simulink library "lib_BuildingThermalTL"  (R2026a)
settings: Solver=VariableStepAuto
libraries: ExternalWall_lib x47, WallSelector_lib x36, fl_lib x20, RoomWithRadiatorAndUFP x15, RoomLevelControl_lib x2
(part 1 of 5)
settings Model: Creator=vikrants  LastModifiedBy=vikrants

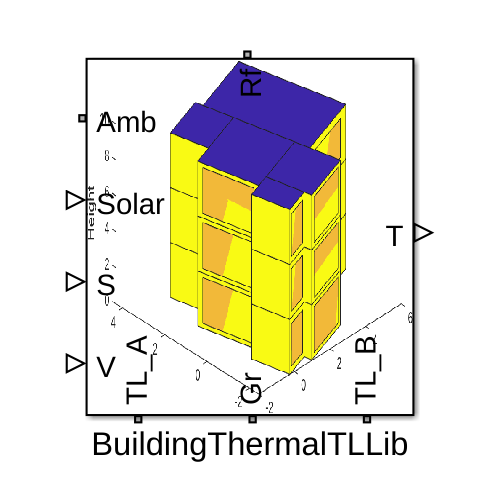
[thumbnail: Simulink's stored preview of the top-level diagram]
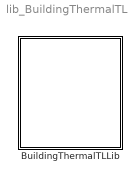
== system lib_BuildingThermalTL ==
  BuildingThermalTLLib : Subsystem
      settings: PortSchema="{\"entries\":[{\"content\":{\"sides\":[{\"content\":{\"connectorIds\":[\"LConn1\",\"LConn2\",\"LConn3\",\"LConn4\"]},\"type\":\"ConnectorPlacement.EquallySpacedRectSide\",\"uuid\":\"7752f6df-96a7-479d-81d0-a1acc354bc8e\"},{\"content\":{\"connectorIds\":[\"RConn1\"],\"side\":\"RIGHT\"},\"type\":\"ConnectorPlacement.EquallySpacedRectSide\",\"uuid\":\"82977a39-da32-427b-b825-91d4f4b46228\"},{\"content\":{\"connectorIds\":[\"LConn5\"],\"side\":\"TOP\"},\"type\":\"ConnectorPlacement.EquallySpacedRectSide\",\"uuid\":\"1009c293-c44e-4703-95e9-5e2b8b92121f\"},{\"content\":{\"connectorIds\":[\"RConn2\",\"RConn3\",\"RConn4\"],\"side\":\"BOTTOM\"},\"type\":\"ConnectorPlacement.EquallySpacedRectSide\",\"uuid\":\"f5115ea0-1536-4578-9315-a120045d60b6\"}]},\"type\":\"ConnectorPlacement.EquallySpacedConnector\",\"uuid\":\"9ddcc19a-e483-4977-a29d-e666927a4fbb\"}],\"packageUris\":[\"http://schema.mathworks.com/mf0/Connector/R2020b\"],\"version\":\"1.0\"}"
      mask Display: image('lib_BuildingThermalTL.png')

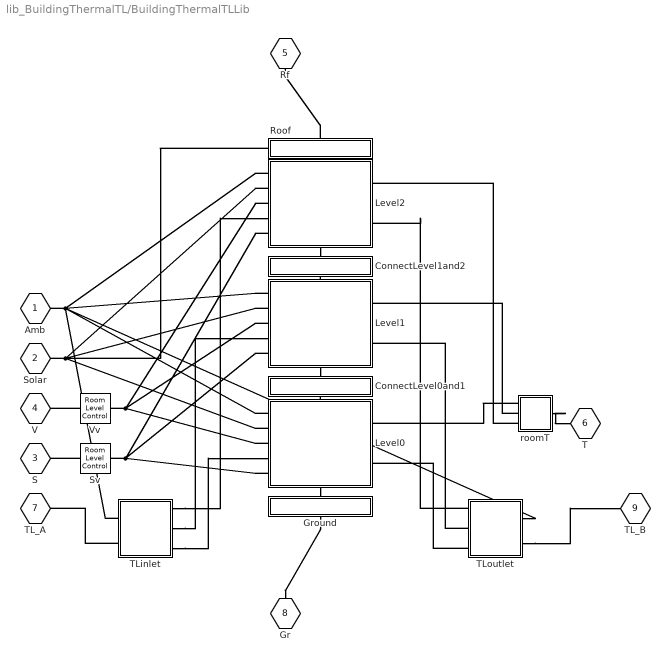
== system lib_BuildingThermalTL/BuildingThermalTLLib ==
  ConnectLevel0and1 : Subsystem
      settings: PortSchema="{\"entries\":[{\"content\":{\"sides\":[{\"content\":{},\"type\":\"ConnectorPlacement.EquallySpacedRectSide\",\"uuid\":\"bfcbcdaf-7e68-43ba-b21b-739e3d917df2\"},{\"content\":{\"side\":\"RIGHT\"},\"type\":\"ConnectorPlacement.EquallySpacedRectSide\",\"uuid\":\"1db46710-465c-454f-9fe4-f8c04c90b155\"},{\"content\":{\"connectorIds\":[\"LConn1\"],\"side\":\"TOP\"},\"type\":\"ConnectorPlacement.EquallySpacedRectSide\",\"uuid\":\"8ba3322a-28ec-4bcd-a32b-78c0e69bc71f\"},{\"content\":{\"connectorIds\":[\"RConn1\"],\"side\":\"BOTTOM\"},\"type\":\"ConnectorPlacement.EquallySpacedRectSide\",\"uuid\":\"deed2508-d6b6-4274-ba05-c274e079ee5b\"}]},\"type\":\"ConnectorPlacement.EquallySpacedConnector\",\"uuid\":\"bc7fd7cc-de66-4685-913a-91b57874b9ec\"}],\"packageUris\":[\"http://schema.mathworks.com/mf0/Connector/R2020b\"],\"version\":\"1.0\"}"
  ConnectLevel1and2 : Subsystem
      settings: PortSchema="{\"entries\":[{\"content\":{\"sides\":[{\"content\":{},\"type\":\"ConnectorPlacement.EquallySpacedRectSide\",\"uuid\":\"bfcbcdaf-7e68-43ba-b21b-739e3d917df2\"},{\"content\":{\"side\":\"RIGHT\"},\"type\":\"ConnectorPlacement.EquallySpacedRectSide\",\"uuid\":\"1db46710-465c-454f-9fe4-f8c04c90b155\"},{\"content\":{\"connectorIds\":[\"LConn1\"],\"side\":\"TOP\"},\"type\":\"ConnectorPlacement.EquallySpacedRectSide\",\"uuid\":\"8ba3322a-28ec-4bcd-a32b-78c0e69bc71f\"},{\"content\":{\"connectorIds\":[\"RConn1\"],\"side\":\"BOTTOM\"},\"type\":\"ConnectorPlacement.EquallySpacedRectSide\",\"uuid\":\"a3884e5a-d735-4cb4-ba23-284eb55af6b2\"}]},\"type\":\"ConnectorPlacement.EquallySpacedConnector\",\"uuid\":\"bc7fd7cc-de66-4685-913a-91b57874b9ec\"}],\"packageUris\":[\"http://schema.mathworks.com/mf0/Connector/R2020b\"],\"version\":\"1.0\"}"
  Ground : Subsystem
      settings: PortSchema="{\"entries\":[{\"content\":{\"sides\":[{\"content\":{},\"type\":\"ConnectorPlacement.EquallySpacedRectSide\",\"uuid\":\"bfcbcdaf-7e68-43ba-b21b-739e3d917df2\"},{\"content\":{\"side\":\"RIGHT\"},\"type\":\"ConnectorPlacement.EquallySpacedRectSide\",\"uuid\":\"1db46710-465c-454f-9fe4-f8c04c90b155\"},{\"content\":{\"connectorIds\":[\"LConn1\"],\"side\":\"TOP\"},\"type\":\"ConnectorPlacement.EquallySpacedRectSide\",\"uuid\":\"8ba3322a-28ec-4bcd-a32b-78c0e69bc71f\"},{\"content\":{\"connectorIds\":[\"RConn1\"],\"side\":\"BOTTOM\"},\"type\":\"ConnectorPlacement.EquallySpacedRectSide\",\"uuid\":\"62f17525-a3e4-4f49-87ca-4f069149a482\"}]},\"type\":\"ConnectorPlacement.EquallySpacedConnector\",\"uuid\":\"bc7fd7cc-de66-4685-913a-91b57874b9ec\"}],\"packageUris\":[\"http://schema.mathworks.com/mf0/Connector/R2020b\"],\"version\":\"1.0\"}"
  Level0 : Subsystem
      settings: PortSchema="{\"entries\":[{\"content\":{\"sides\":[{\"content\":{\"connectorIds\":[\"LConn1\",\"LConn2\",\"LConn3\",\"LConn4\",\"LConn5\"]},\"type\":\"ConnectorPlacement.EquallySpacedRectSide\",\"uuid\":\"deabb5b8-c24f-48fb-93fe-496ddd92a6f5\"},{\"content\":{\"connectorIds\":[\"RConn1\",\"RConn2\"],\"side\":\"RIGHT\"},\"type\":\"ConnectorPlacement.EquallySpacedRectSide\",\"uuid\":\"554b1cd5-3627-4990-b424-868f4b09881c\"},{\"content\":{\"connectorIds\":[\"LConn6\"],\"side\":\"TOP\"},\"type\":\"ConnectorPlacement.EquallySpacedRectSide\",\"uuid\":\"21e43258-e745-4398-91f3-d3fef9b84a06\"},{\"content\":{\"connectorIds\":[\"RConn3\"],\"side\":\"BOTTOM\"},\"type\":\"ConnectorPlacement.EquallySpacedRectSide\",\"uuid\":\"c4a37077-5805-4bd2-bf9a-83a9fce6d671\"}]},\"type\":\"ConnectorPlacement.EquallySpacedConnector\",\"uuid\":\"65daea52-a8f7-4065-b13d-a48c2b26414b\"}],\"packageUris\":[\"http://schema.mathworks.com/mf0/Connector/R2020b\"],\"version\":\"1.0\"}"
  Level1 : Subsystem
      settings: PortSchema="{\"entries\":[{\"content\":{\"sides\":[{\"content\":{\"connectorIds\":[\"LConn1\",\"LConn2\",\"LConn3\",\"LConn4\",\"LConn5\"]},\"type\":\"ConnectorPlacement.EquallySpacedRectSide\",\"uuid\":\"deabb5b8-c24f-48fb-93fe-496ddd92a6f5\"},{\"content\":{\"connectorIds\":[\"RConn1\",\"RConn2\"],\"side\":\"RIGHT\"},\"type\":\"ConnectorPlacement.EquallySpacedRectSide\",\"uuid\":\"554b1cd5-3627-4990-b424-868f4b09881c\"},{\"content\":{\"connectorIds\":[\"LConn6\"],\"side\":\"TOP\"},\"type\":\"ConnectorPlacement.EquallySpacedRectSide\",\"uuid\":\"21e43258-e745-4398-91f3-d3fef9b84a06\"},{\"content\":{\"connectorIds\":[\"RConn3\"],\"side\":\"BOTTOM\"},\"type\":\"ConnectorPlacement.EquallySpacedRectSide\",\"uuid\":\"0cd4818a-d5ce-48ab-9e4b-3620ed85a804\"}]},\"type\":\"ConnectorPlacement.EquallySpacedConnector\",\"uuid\":\"65daea52-a8f7-4065-b13d-a48c2b26414b\"}],\"packageUris\":[\"http://schema.mathworks.com/mf0/Connector/R2020b\"],\"version\":\"1.0\"}"
  Level2 : Subsystem
      settings: PortSchema="{\"entries\":[{\"content\":{\"sides\":[{\"content\":{\"connectorIds\":[\"LConn1\",\"LConn2\",\"LConn3\",\"LConn4\",\"LConn5\"]},\"type\":\"ConnectorPlacement.EquallySpacedRectSide\",\"uuid\":\"deabb5b8-c24f-48fb-93fe-496ddd92a6f5\"},{\"content\":{\"connectorIds\":[\"RConn1\",\"RConn2\"],\"side\":\"RIGHT\"},\"type\":\"ConnectorPlacement.EquallySpacedRectSide\",\"uuid\":\"554b1cd5-3627-4990-b424-868f4b09881c\"},{\"content\":{\"connectorIds\":[\"LConn6\"],\"side\":\"TOP\"},\"type\":\"ConnectorPlacement.EquallySpacedRectSide\",\"uuid\":\"21e43258-e745-4398-91f3-d3fef9b84a06\"},{\"content\":{\"connectorIds\":[\"RConn3\"],\"side\":\"BOTTOM\"},\"type\":\"ConnectorPlacement.EquallySpacedRectSide\",\"uuid\":\"b1810ee7-4d08-40c9-8b26-724c07e39c34\"}]},\"type\":\"ConnectorPlacement.EquallySpacedConnector\",\"uuid\":\"65daea52-a8f7-4065-b13d-a48c2b26414b\"}],\"packageUris\":[\"http://schema.mathworks.com/mf0/Connector/R2020b\"],\"version\":\"1.0\"}"
  Roof : Subsystem
      settings: PortSchema="{\"entries\":[{\"content\":{\"sides\":[{\"content\":{\"connectorIds\":[\"LConn1\"]},\"type\":\"ConnectorPlacement.EquallySpacedRectSide\",\"uuid\":\"330a1f4c-788b-45d3-8144-461e13e4bc2b\"},{\"content\":{\"side\":\"RIGHT\"},\"type\":\"ConnectorPlacement.EquallySpacedRectSide\",\"uuid\":\"2ff68f0e-d161-486d-a47e-10633b293a9f\"},{\"content\":{\"connectorIds\":[\"LConn2\"],\"side\":\"TOP\"},\"type\":\"ConnectorPlacement.EquallySpacedRectSide\",\"uuid\":\"a18254b5-007e-4575-8004-ea2058ac2122\"},{\"content\":{\"connectorIds\":[\"RConn1\"],\"side\":\"BOTTOM\"},\"type\":\"ConnectorPlacement.EquallySpacedRectSide\",\"uuid\":\"b51dbafe-ebd1-4fa9-aca1-0d2d3d6d1c44\"}]},\"type\":\"ConnectorPlacement.EquallySpacedConnector\",\"uuid\":\"c0f19b20-ad71-4ed9-8cf3-6c486454730f\"}],\"packageUris\":[\"http://schema.mathworks.com/mf0/Connector/R2020b\"],\"version\":\"1.0\"}"
  Sv : RoomLevelControl_lib/Room Level Control  portOption=roomControlOption.heat  roomMapping=[1 1 1 1;1 1 2 2;1 1 3 3;1 1 4 4;1 1 5 5;2 2 1 6;2 2 2 7;2 2 3 8;2 2 4 9;2 2 5 10;3 3 1 11;3 3 2 12;3 3 3 13;3 3 4 14;3 3 5 15]
  TLinlet : Subsystem
  TLoutlet : Subsystem
  Vv : RoomLevelControl_lib/Room Level Control  portOption=roomControlOption.valve  roomMapping=[1 1 1 1;1 1 2 2;1 1 3 3;1 1 4 4;1 1 5 5;2 2 1 6;2 2 2 7;2 2 3 8;2 2 4 9;2 2 5 10;3 3 1 11;3 3 2 12;3 3 3 13;3 3 4 14;3 3 5 15]
  roomT : Subsystem
  Amb : PMIOPort  Side=Left
  Solar : PMIOPort  Port=2  Side=Left
  S : PMIOPort  Port=3  Side=Left
  V : PMIOPort  Port=4  Side=Left
  Rf : PMIOPort  Port=5  Side=Left
  T : PMIOPort  Port=6  Side=Right
  TL_A : PMIOPort  Port=7  Side=Right
  Gr : PMIOPort  Port=8  Side=Right
  TL_B : PMIOPort  Port=9  Side=Right
  connections:
  TLinlet/RConn1 -- Level2/LConn4
  TLoutlet/LConn1 -- Level2/RConn2
  TLinlet/RConn2 -- Level1/LConn4
  TLoutlet/LConn2 -- Level1/RConn2
  TLinlet/RConn3 -- Level0/LConn4
  TLoutlet/LConn3 -- Level0/RConn2
  Level0/RConn3 -- Ground/LConn1
  Level1/RConn3 -- ConnectLevel0and1/LConn1
  Level0/LConn6 -- ConnectLevel0and1/RConn1
  Level2/RConn3 -- ConnectLevel1and2/LConn1
  Level1/LConn6 -- ConnectLevel1and2/RConn1
  Level2/LConn6 -- Roof/RConn1
  Sv/LConn1 -- S/RConn1
  Vv/LConn1 -- V/RConn1
  Roof/LConn2 -- Rf/RConn1
  Ground/RConn1 -- Gr/RConn1
  Roof/LConn1 -- Level0/LConn2 -- Level1/LConn2 -- Solar/RConn1 -- Level2/LConn2
  Level0/LConn1 -- Level1/LConn1 -- Level2/LConn1 -- TLinlet/LConn1 -- Amb/RConn1 -- TLoutlet/RConn1
  Level0/LConn3 -- Level1/LConn3 -- Vv/RConn1 -- Level2/LConn3
  Level0/LConn5 -- Level1/LConn5 -- Sv/RConn1 -- Level2/LConn5
  TLinlet/LConn2 -- TL_A/RConn1
  TLoutlet/RConn2 -- TL_B/RConn1
  roomT/LConn1 -- Level0/RConn1
  roomT/LConn2 -- Level1/RConn1
  roomT/LConn3 -- Level2/RConn1
  roomT/RConn1 -- T/RConn1

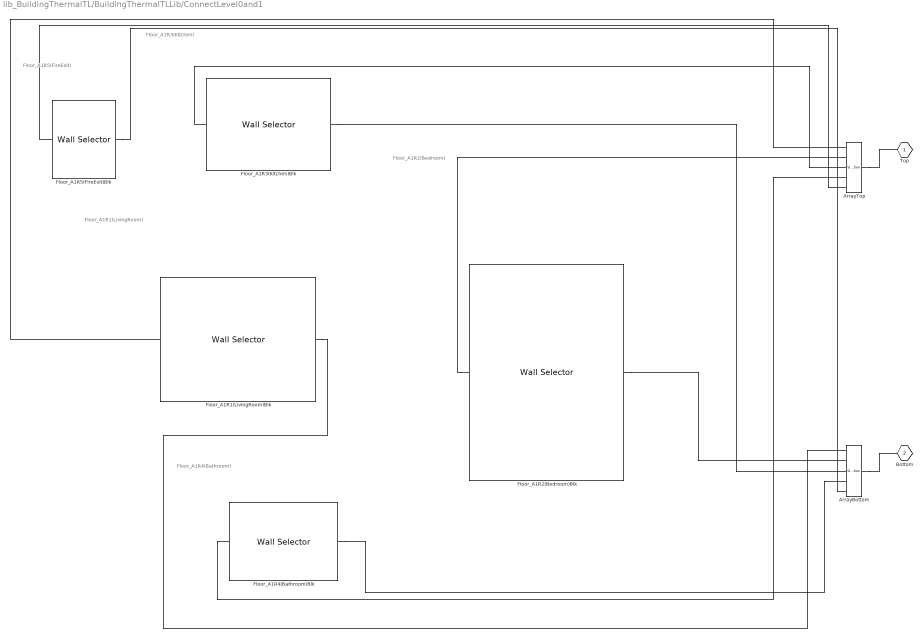
== system lib_BuildingThermalTL/BuildingThermalTLLib/ConnectLevel0and1 ==
  note: Floor_A1R1(LivingRoom)
  note: Floor_A1R2(Bedroom)
  note: Floor_A1R3(Kitchen)
  note: Floor_A1R4(Bathroom)
  note: Floor_A1R5(FireExit)
  ArrayBottom : SimscapeArrayConnection  Domain=foundation.thermal.thermal  ConcatenateDimension=1  NumScalarElements=5
  ArrayTop : SimscapeArrayConnection  Domain=foundation.thermal.thermal  ConcatenateDimension=1  NumScalarElements=5
  Floor_A1R1(LivingRoom)Blk : WallSelector_lib/Wall Selector  optWall=wallModelOption.wallOnly  wallLength=2.4384 % Parameterized on : 14-Jun-2026 15:20:36 m  wallHeight=3.048 % Parameterized on : 14-Jun-2026 15:20:36 m  wallThickness=0.03 % Parameterized on : 14-Jun-2026 15:20:36 m  wallMaterialDen=1400 % Parameterized on : 14-Jun-2026 15:20:39 kg/m^3  wallMaterialCp=1000 % Parameterized on : 14-Jun-2026 15:20:39 J/(K*kg)  wallAbsorptivity=0.5  wallThermalK=0.7 % Parameterized on : 14-Jun-2026 15:20:39 W/(K*m)  winLength=1 m  winHeight=0.5 m  winThickness=0.007 m  winMaterialDen=2500 kg/m^3  winMaterialCp=787 J/(K*kg)  winAbsorptivity=0.35  winThermalK=1 W/(K*m)  winTransmissivity=0.45  ventLength=0.1 m  ventHeight=0.1 m  extToWallHTC=30 % Parameterized on : 14-Jun-2026 15:20:39 W/(K*m^2)  intToRoomHTC=30 % Parameterized on : 14-Jun-2026 15:20:39 W/(K*m^2)  iniT=300 % Parameterized on : 14-Jun-2026 15:20:39 K
  Floor_A1R2(Bedroom)Blk : WallSelector_lib/Wall Selector  optWall=wallModelOption.wallOnly  wallLength=4.2672 % Parameterized on : 14-Jun-2026 15:20:36 m  wallHeight=3.048 % Parameterized on : 14-Jun-2026 15:20:36 m  wallThickness=0.03 % Parameterized on : 14-Jun-2026 15:20:36 m  wallMaterialDen=1400 % Parameterized on : 14-Jun-2026 15:20:39 kg/m^3  wallMaterialCp=1000 % Parameterized on : 14-Jun-2026 15:20:39 J/(K*kg)  wallAbsorptivity=0.5  wallThermalK=0.7 % Parameterized on : 14-Jun-2026 15:20:39 W/(K*m)  winLength=1 m  winHeight=0.5 m  winThickness=0.007 m  winMaterialDen=2500 kg/m^3  winMaterialCp=787 J/(K*kg)  winAbsorptivity=0.35  winThermalK=1 W/(K*m)  winTransmissivity=0.45  ventLength=0.1 m  ventHeight=0.1 m  extToWallHTC=30 % Parameterized on : 14-Jun-2026 15:20:39 W/(K*m^2)  intToRoomHTC=30 % Parameterized on : 14-Jun-2026 15:20:39 W/(K*m^2)  iniT=300 % Parameterized on : 14-Jun-2026 15:20:39 K
  Floor_A1R3(Kitchen)Blk : WallSelector_lib/Wall Selector  optWall=wallModelOption.wallOnly  wallLength=1.8288 % Parameterized on : 14-Jun-2026 15:20:36 m  wallHeight=2.4384 % Parameterized on : 14-Jun-2026 15:20:36 m  wallThickness=0.03 % Parameterized on : 14-Jun-2026 15:20:36 m  wallMaterialDen=1400 % Parameterized on : 14-Jun-2026 15:20:39 kg/m^3  wallMaterialCp=1000 % Parameterized on : 14-Jun-2026 15:20:39 J/(K*kg)  wallAbsorptivity=0.5  wallThermalK=0.7 % Parameterized on : 14-Jun-2026 15:20:39 W/(K*m)  winLength=1 m  winHeight=0.5 m  winThickness=0.007 m  winMaterialDen=2500 kg/m^3  winMaterialCp=787 J/(K*kg)  winAbsorptivity=0.35  winThermalK=1 W/(K*m)  winTransmissivity=0.45  ventLength=0.1 m  ventHeight=0.1 m  extToWallHTC=30 % Parameterized on : 14-Jun-2026 15:20:39 W/(K*m^2)  intToRoomHTC=30 % Parameterized on : 14-Jun-2026 15:20:39 W/(K*m^2)  iniT=300 % Parameterized on : 14-Jun-2026 15:20:39 K
  Floor_A1R4(Bathroom)Blk : WallSelector_lib/Wall Selector  optWall=wallModelOption.wallOnly  wallLength=1.524 % Parameterized on : 14-Jun-2026 15:20:36 m  wallHeight=2.1336 % Parameterized on : 14-Jun-2026 15:20:36 m  wallThickness=0.03 % Parameterized on : 14-Jun-2026 15:20:36 m  wallMaterialDen=1400 % Parameterized on : 14-Jun-2026 15:20:39 kg/m^3  wallMaterialCp=1000 % Parameterized on : 14-Jun-2026 15:20:39 J/(K*kg)  wallAbsorptivity=0.5  wallThermalK=0.7 % Parameterized on : 14-Jun-2026 15:20:39 W/(K*m)  winLength=1 m  winHeight=0.5 m  winThickness=0.007 m  winMaterialDen=2500 kg/m^3  winMaterialCp=787 J/(K*kg)  winAbsorptivity=0.35  winThermalK=1 W/(K*m)  winTransmissivity=0.45  ventLength=0.1 m  ventHeight=0.1 m  extToWallHTC=30 % Parameterized on : 14-Jun-2026 15:20:39 W/(K*m^2)  intToRoomHTC=30 % Parameterized on : 14-Jun-2026 15:20:39 W/(K*m^2)  iniT=300 % Parameterized on : 14-Jun-2026 15:20:39 K
  Floor_A1R5(FireExit)Blk : WallSelector_lib/Wall Selector  optWall=wallModelOption.wallOnly  wallLength=1.524 % Parameterized on : 14-Jun-2026 15:20:36 m  wallHeight=1.2192 % Parameterized on : 14-Jun-2026 15:20:36 m  wallThickness=0.03 % Parameterized on : 14-Jun-2026 15:20:36 m  wallMaterialDen=1400 % Parameterized on : 14-Jun-2026 15:20:39 kg/m^3  wallMaterialCp=1000 % Parameterized on : 14-Jun-2026 15:20:39 J/(K*kg)  wallAbsorptivity=0.5  wallThermalK=0.7 % Parameterized on : 14-Jun-2026 15:20:39 W/(K*m)  winLength=1 m  winHeight=0.5 m  winThickness=0.007 m  winMaterialDen=2500 kg/m^3  winMaterialCp=787 J/(K*kg)  winAbsorptivity=0.35  winThermalK=1 W/(K*m)  winTransmissivity=0.45  ventLength=0.1 m  ventHeight=0.1 m  extToWallHTC=30 % Parameterized on : 14-Jun-2026 15:20:39 W/(K*m^2)  intToRoomHTC=30 % Parameterized on : 14-Jun-2026 15:20:39 W/(K*m^2)  iniT=300 % Parameterized on : 14-Jun-2026 15:20:39 K
  Top : PMIOPort  Side=Left
  Bottom : PMIOPort  Port=2  Side=Right
  connections:
  ArrayTop/RConn1 -- Top/RConn1
  Floor_A1R1(LivingRoom)Blk/LConn1 -- ArrayTop/LConn1
  Floor_A1R2(Bedroom)Blk/LConn1 -- ArrayTop/LConn2
  Floor_A1R3(Kitchen)Blk/LConn1 -- ArrayTop/LConn3
  Floor_A1R4(Bathroom)Blk/LConn1 -- ArrayTop/LConn4
  Floor_A1R5(FireExit)Blk/LConn1 -- ArrayTop/LConn5
  ArrayBottom/RConn1 -- Bottom/RConn1
  Floor_A1R1(LivingRoom)Blk/RConn1 -- ArrayBottom/LConn1
  Floor_A1R2(Bedroom)Blk/RConn1 -- ArrayBottom/LConn2
  Floor_A1R3(Kitchen)Blk/RConn1 -- ArrayBottom/LConn3
  Floor_A1R4(Bathroom)Blk/RConn1 -- ArrayBottom/LConn4
  Floor_A1R5(FireExit)Blk/RConn1 -- ArrayBottom/LConn5

== system lib_BuildingThermalTL/BuildingThermalTLLib/ConnectLevel1and2 ==
  note: Floor_A2R1(LivingRoom)
  note: Floor_A2R2(Bedroom)
  note: Floor_A2R3(Kitchen)
  note: Floor_A2R4(Bathroom)
  note: Floor_A2R5(FireExit)
  ArrayBottom : SimscapeArrayConnection  Domain=foundation.thermal.thermal  ConcatenateDimension=1  NumScalarElements=5
  ArrayTop : SimscapeArrayConnection  Domain=foundation.thermal.thermal  ConcatenateDimension=1  NumScalarElements=5
  Floor_A2R1(LivingRoom)Blk : WallSelector_lib/Wall Selector  optWall=wallModelOption.wallOnly  wallLength=2.4384 % Parameterized on : 14-Jun-2026 15:20:36 m  wallHeight=3.048 % Parameterized on : 14-Jun-2026 15:20:36 m  wallThickness=0.03 % Parameterized on : 14-Jun-2026 15:20:36 m  wallMaterialDen=1400 % Parameterized on : 14-Jun-2026 15:20:39 kg/m^3  wallMaterialCp=1000 % Parameterized on : 14-Jun-2026 15:20:39 J/(K*kg)  wallAbsorptivity=0.5  wallThermalK=0.7 % Parameterized on : 14-Jun-2026 15:20:39 W/(K*m)  winLength=1 m  winHeight=0.5 m  winThickness=0.007 m  winMaterialDen=2500 kg/m^3  winMaterialCp=787 J/(K*kg)  winAbsorptivity=0.35  winThermalK=1 W/(K*m)  winTransmissivity=0.45  ventLength=0.1 m  ventHeight=0.1 m  extToWallHTC=30 % Parameterized on : 14-Jun-2026 15:20:39 W/(K*m^2)  intToRoomHTC=30 % Parameterized on : 14-Jun-2026 15:20:39 W/(K*m^2)  iniT=300 % Parameterized on : 14-Jun-2026 15:20:39 K
  Floor_A2R2(Bedroom)Blk : WallSelector_lib/Wall Selector  optWall=wallModelOption.wallOnly  wallLength=4.2672 % Parameterized on : 14-Jun-2026 15:20:36 m  wallHeight=3.048 % Parameterized on : 14-Jun-2026 15:20:36 m  wallThickness=0.03 % Parameterized on : 14-Jun-2026 15:20:36 m  wallMaterialDen=1400 % Parameterized on : 14-Jun-2026 15:20:39 kg/m^3  wallMaterialCp=1000 % Parameterized on : 14-Jun-2026 15:20:39 J/(K*kg)  wallAbsorptivity=0.5  wallThermalK=0.7 % Parameterized on : 14-Jun-2026 15:20:39 W/(K*m)  winLength=1 m  winHeight=0.5 m  winThickness=0.007 m  winMaterialDen=2500 kg/m^3  winMaterialCp=787 J/(K*kg)  winAbsorptivity=0.35  winThermalK=1 W/(K*m)  winTransmissivity=0.45  ventLength=0.1 m  ventHeight=0.1 m  extToWallHTC=30 % Parameterized on : 14-Jun-2026 15:20:39 W/(K*m^2)  intToRoomHTC=30 % Parameterized on : 14-Jun-2026 15:20:39 W/(K*m^2)  iniT=300 % Parameterized on : 14-Jun-2026 15:20:39 K
  Floor_A2R3(Kitchen)Blk : WallSelector_lib/Wall Selector  optWall=wallModelOption.wallOnly  wallLength=1.8288 % Parameterized on : 14-Jun-2026 15:20:36 m  wallHeight=2.4384 % Parameterized on : 14-Jun-2026 15:20:36 m  wallThickness=0.03 % Parameterized on : 14-Jun-2026 15:20:36 m  wallMaterialDen=1400 % Parameterized on : 14-Jun-2026 15:20:39 kg/m^3  wallMaterialCp=1000 % Parameterized on : 14-Jun-2026 15:20:39 J/(K*kg)  wallAbsorptivity=0.5  wallThermalK=0.7 % Parameterized on : 14-Jun-2026 15:20:39 W/(K*m)  winLength=1 m  winHeight=0.5 m  winThickness=0.007 m  winMaterialDen=2500 kg/m^3  winMaterialCp=787 J/(K*kg)  winAbsorptivity=0.35  winThermalK=1 W/(K*m)  winTransmissivity=0.45  ventLength=0.1 m  ventHeight=0.1 m  extToWallHTC=30 % Parameterized on : 14-Jun-2026 15:20:39 W/(K*m^2)  intToRoomHTC=30 % Parameterized on : 14-Jun-2026 15:20:39 W/(K*m^2)  iniT=300 % Parameterized on : 14-Jun-2026 15:20:39 K
  Floor_A2R4(Bathroom)Blk : WallSelector_lib/Wall Selector  optWall=wallModelOption.wallOnly  wallLength=1.524 % Parameterized on : 14-Jun-2026 15:20:36 m  wallHeight=2.1336 % Parameterized on : 14-Jun-2026 15:20:36 m  wallThickness=0.03 % Parameterized on : 14-Jun-2026 15:20:36 m  wallMaterialDen=1400 % Parameterized on : 14-Jun-2026 15:20:39 kg/m^3  wallMaterialCp=1000 % Parameterized on : 14-Jun-2026 15:20:39 J/(K*kg)  wallAbsorptivity=0.5  wallThermalK=0.7 % Parameterized on : 14-Jun-2026 15:20:39 W/(K*m)  winLength=1 m  winHeight=0.5 m  winThickness=0.007 m  winMaterialDen=2500 kg/m^3  winMaterialCp=787 J/(K*kg)  winAbsorptivity=0.35  winThermalK=1 W/(K*m)  winTransmissivity=0.45  ventLength=0.1 m  ventHeight=0.1 m  extToWallHTC=30 % Parameterized on : 14-Jun-2026 15:20:39 W/(K*m^2)  intToRoomHTC=30 % Parameterized on : 14-Jun-2026 15:20:39 W/(K*m^2)  iniT=300 % Parameterized on : 14-Jun-2026 15:20:39 K
  Floor_A2R5(FireExit)Blk : WallSelector_lib/Wall Selector  optWall=wallModelOption.wallOnly  wallLength=1.524 % Parameterized on : 14-Jun-2026 15:20:36 m  wallHeight=1.2192 % Parameterized on : 14-Jun-2026 15:20:36 m  wallThickness=0.03 % Parameterized on : 14-Jun-2026 15:20:36 m  wallMaterialDen=1400 % Parameterized on : 14-Jun-2026 15:20:39 kg/m^3  wallMaterialCp=1000 % Parameterized on : 14-Jun-2026 15:20:39 J/(K*kg)  wallAbsorptivity=0.5  wallThermalK=0.7 % Parameterized on : 14-Jun-2026 15:20:39 W/(K*m)  winLength=1 m  winHeight=0.5 m  winThickness=0.007 m  winMaterialDen=2500 kg/m^3  winMaterialCp=787 J/(K*kg)  winAbsorptivity=0.35  winThermalK=1 W/(K*m)  winTransmissivity=0.45  ventLength=0.1 m  ventHeight=0.1 m  extToWallHTC=30 % Parameterized on : 14-Jun-2026 15:20:39 W/(K*m^2)  intToRoomHTC=30 % Parameterized on : 14-Jun-2026 15:20:39 W/(K*m^2)  iniT=300 % Parameterized on : 14-Jun-2026 15:20:39 K
  Top : PMIOPort  Side=Left
  Bottom : PMIOPort  Port=2  Side=Right
  connections:
  ArrayTop/RConn1 -- Top/RConn1
  Floor_A2R1(LivingRoom)Blk/LConn1 -- ArrayTop/LConn1
  Floor_A2R2(Bedroom)Blk/LConn1 -- ArrayTop/LConn2
  Floor_A2R3(Kitchen)Blk/LConn1 -- ArrayTop/LConn3
  Floor_A2R4(Bathroom)Blk/LConn1 -- ArrayTop/LConn4
  Floor_A2R5(FireExit)Blk/LConn1 -- ArrayTop/LConn5
  ArrayBottom/RConn1 -- Bottom/RConn1
  Floor_A2R1(LivingRoom)Blk/RConn1 -- ArrayBottom/LConn1
  Floor_A2R2(Bedroom)Blk/RConn1 -- ArrayBottom/LConn2
  Floor_A2R3(Kitchen)Blk/RConn1 -- ArrayBottom/LConn3
  Floor_A2R4(Bathroom)Blk/RConn1 -- ArrayBottom/LConn4
  Floor_A2R5(FireExit)Blk/RConn1 -- ArrayBottom/LConn5

== system lib_BuildingThermalTL/BuildingThermalTLLib/Ground ==
  note: Ground_A1R1(LivingRoom)
  note: Ground_A1R2(Bedroom)
  note: Ground_A1R3(Kitchen)
  note: Ground_A1R4(Bathroom)
  note: Ground_A1R5(FireExit)
  ArrayBottom : SimscapeArrayConnection  Domain=foundation.thermal.thermal  ConcatenateDimension=1  NumScalarElements=5
  ArrayTop : SimscapeArrayConnection  Domain=foundation.thermal.thermal  ConcatenateDimension=1  NumScalarElements=5
  Ground_A1R1(LivingRoom)Blk : WallSelector_lib/Wall Selector  optWall=wallModelOption.wallOnly  wallLength=2.4384 % Parameterized on : 14-Jun-2026 15:20:36 m  wallHeight=3.048 % Parameterized on : 14-Jun-2026 15:20:36 m  wallThickness=0.03 % Parameterized on : 14-Jun-2026 15:20:36 m  wallMaterialDen=1400 % Parameterized on : 14-Jun-2026 15:20:39 kg/m^3  wallMaterialCp=1000 % Parameterized on : 14-Jun-2026 15:20:39 J/(K*kg)  wallAbsorptivity=0.5  wallThermalK=0.7 % Parameterized on : 14-Jun-2026 15:20:39 W/(K*m)  winLength=1 m  winHeight=0.5 m  winThickness=0.007 m  winMaterialDen=2500 kg/m^3  winMaterialCp=787 J/(K*kg)  winAbsorptivity=0.35  winThermalK=1 W/(K*m)  winTransmissivity=0.45  ventLength=0.1 m  ventHeight=0.1 m  extToWallHTC=30 % Parameterized on : 14-Jun-2026 15:20:39 W/(K*m^2)  intToRoomHTC=30 % Parameterized on : 14-Jun-2026 15:20:39 W/(K*m^2)  iniT=300 % Parameterized on : 14-Jun-2026 15:20:39 K
  Ground_A1R2(Bedroom)Blk : WallSelector_lib/Wall Selector  optWall=wallModelOption.wallOnly  wallLength=4.2672 % Parameterized on : 14-Jun-2026 15:20:36 m  wallHeight=3.048 % Parameterized on : 14-Jun-2026 15:20:36 m  wallThickness=0.03 % Parameterized on : 14-Jun-2026 15:20:36 m  wallMaterialDen=1400 % Parameterized on : 14-Jun-2026 15:20:39 kg/m^3  wallMaterialCp=1000 % Parameterized on : 14-Jun-2026 15:20:39 J/(K*kg)  wallAbsorptivity=0.5  wallThermalK=0.7 % Parameterized on : 14-Jun-2026 15:20:39 W/(K*m)  winLength=1 m  winHeight=0.5 m  winThickness=0.007 m  winMaterialDen=2500 kg/m^3  winMaterialCp=787 J/(K*kg)  winAbsorptivity=0.35  winThermalK=1 W/(K*m)  winTransmissivity=0.45  ventLength=0.1 m  ventHeight=0.1 m  extToWallHTC=30 % Parameterized on : 14-Jun-2026 15:20:39 W/(K*m^2)  intToRoomHTC=30 % Parameterized on : 14-Jun-2026 15:20:39 W/(K*m^2)  iniT=300 % Parameterized on : 14-Jun-2026 15:20:39 K
  Ground_A1R3(Kitchen)Blk : WallSelector_lib/Wall Selector  optWall=wallModelOption.wallOnly  wallLength=1.8288 % Parameterized on : 14-Jun-2026 15:20:36 m  wallHeight=2.4384 % Parameterized on : 14-Jun-2026 15:20:36 m  wallThickness=0.03 % Parameterized on : 14-Jun-2026 15:20:36 m  wallMaterialDen=1400 % Parameterized on : 14-Jun-2026 15:20:39 kg/m^3  wallMaterialCp=1000 % Parameterized on : 14-Jun-2026 15:20:39 J/(K*kg)  wallAbsorptivity=0.5  wallThermalK=0.7 % Parameterized on : 14-Jun-2026 15:20:39 W/(K*m)  winLength=1 m  winHeight=0.5 m  winThickness=0.007 m  winMaterialDen=2500 kg/m^3  winMaterialCp=787 J/(K*kg)  winAbsorptivity=0.35  winThermalK=1 W/(K*m)  winTransmissivity=0.45  ventLength=0.1 m  ventHeight=0.1 m  extToWallHTC=30 % Parameterized on : 14-Jun-2026 15:20:39 W/(K*m^2)  intToRoomHTC=30 % Parameterized on : 14-Jun-2026 15:20:39 W/(K*m^2)  iniT=300 % Parameterized on : 14-Jun-2026 15:20:39 K
  Ground_A1R4(Bathroom)Blk : WallSelector_lib/Wall Selector  optWall=wallModelOption.wallOnly  wallLength=1.524 % Parameterized on : 14-Jun-2026 15:20:36 m  wallHeight=2.1336 % Parameterized on : 14-Jun-2026 15:20:36 m  wallThickness=0.03 % Parameterized on : 14-Jun-2026 15:20:36 m  wallMaterialDen=1400 % Parameterized on : 14-Jun-2026 15:20:39 kg/m^3  wallMaterialCp=1000 % Parameterized on : 14-Jun-2026 15:20:39 J/(K*kg)  wallAbsorptivity=0.5  wallThermalK=0.7 % Parameterized on : 14-Jun-2026 15:20:39 W/(K*m)  winLength=1 m  winHeight=0.5 m  winThickness=0.007 m  winMaterialDen=2500 kg/m^3  winMaterialCp=787 J/(K*kg)  winAbsorptivity=0.35  winThermalK=1 W/(K*m)  winTransmissivity=0.45  ventLength=0.1 m  ventHeight=0.1 m  extToWallHTC=30 % Parameterized on : 14-Jun-2026 15:20:39 W/(K*m^2)  intToRoomHTC=30 % Parameterized on : 14-Jun-2026 15:20:39 W/(K*m^2)  iniT=300 % Parameterized on : 14-Jun-2026 15:20:39 K
  Ground_A1R5(FireExit)Blk : WallSelector_lib/Wall Selector  optWall=wallModelOption.wallOnly  wallLength=1.524 % Parameterized on : 14-Jun-2026 15:20:36 m  wallHeight=1.2192 % Parameterized on : 14-Jun-2026 15:20:36 m  wallThickness=0.03 % Parameterized on : 14-Jun-2026 15:20:36 m  wallMaterialDen=1400 % Parameterized on : 14-Jun-2026 15:20:39 kg/m^3  wallMaterialCp=1000 % Parameterized on : 14-Jun-2026 15:20:39 J/(K*kg)  wallAbsorptivity=0.5  wallThermalK=0.7 % Parameterized on : 14-Jun-2026 15:20:39 W/(K*m)  winLength=1 m  winHeight=0.5 m  winThickness=0.007 m  winMaterialDen=2500 kg/m^3  winMaterialCp=787 J/(K*kg)  winAbsorptivity=0.35  winThermalK=1 W/(K*m)  winTransmissivity=0.45  ventLength=0.1 m  ventHeight=0.1 m  extToWallHTC=30 % Parameterized on : 14-Jun-2026 15:20:39 W/(K*m^2)  intToRoomHTC=30 % Parameterized on : 14-Jun-2026 15:20:39 W/(K*m^2)  iniT=300 % Parameterized on : 14-Jun-2026 15:20:39 K
  Top : PMIOPort  Side=Left
  Bottom : PMIOPort  Port=2  Side=Right
  connections:
  ArrayTop/RConn1 -- Top/RConn1
  Ground_A1R1(LivingRoom)Blk/LConn1 -- ArrayTop/LConn1
  Ground_A1R2(Bedroom)Blk/LConn1 -- ArrayTop/LConn2
  Ground_A1R3(Kitchen)Blk/LConn1 -- ArrayTop/LConn3
  Ground_A1R4(Bathroom)Blk/LConn1 -- ArrayTop/LConn4
  Ground_A1R5(FireExit)Blk/LConn1 -- ArrayTop/LConn5
  ArrayBottom/RConn1 -- Bottom/RConn1
  Ground_A1R1(LivingRoom)Blk/RConn1 -- ArrayBottom/LConn1
  Ground_A1R2(Bedroom)Blk/RConn1 -- ArrayBottom/LConn2
  Ground_A1R3(Kitchen)Blk/RConn1 -- ArrayBottom/LConn3
  Ground_A1R4(Bathroom)Blk/RConn1 -- ArrayBottom/LConn4
  Ground_A1R5(FireExit)Blk/RConn1 -- ArrayBottom/LConn5
